simulink library "ddm"  (R2021b)
settings: Solver=VariableStepAuto  StartTime=0.0  StopTime=10.0  RelTol=1e-3
undefined symbols (not defined in the file): ADDM_FrTMTqDev_X_Nm, ADDM_RrTMTqDev_X_Nm, ENUM_ADASACCSTA_ERROR, ENUM_ADASACCSTA_OFF, ENUM_ADASACCSTA_STANDBY, ENUM_ALLOWMOV_ALLOWREADY, ENUM_APS, ENUM_BRKSTA_ERROR, ENUM_BRKSTA_OFF, ENUM_BRKSTA_ON, ENUM_BRKSW_INVALID, ENUM_BRKSW_OFF, ENUM_BRKSW_ON, ENUM_CHGPREACTERRSTA_OBCPRE, ENUM_DCDCFAULTSTA_ANYFAULTLV1, ENUM_DCDCFAULTSTA_ANYFAULTLV2, ENUM_DRIVETRAIN_AWD, ENUM_DRIVETRAIN_FWD, ENUM_DRIVETRAIN_RWD, ENUM_EDUDRTSTA_NORMAL, ENUM_EPBERROR_FAILED, ENUM_EPBSTA_APPLIED, ENUM_EPBSTA_RELEASED, ENUM_ESCAPSSta_APSUNAVAILABLE, ENUM_GEARACTUALPOSN_INVALID, ENUM_GEARACTUALPOSN_P, ENUM_HVBATTREADYPRE_READY, ENUM_HWRESETSTA_HWRESETING, ENUM_MCUWARN_LV0, ENUM_MCUWARN_LV1, ENUM_MCUWARN_LV2, ENUM_MCUWARN_LV3, ENUM_MCUWARN_NOERROR, ENUM_OBCFAULTSTA_ANYFAULT, ENUM_PAS_R2F2, ENUM_PDFAULT_BATTPDFAIL, ENUM_PDFAULT_DCDCDISABLE, ENUM_PDFAULT_MCUDISABLE, ENUM_PDFAULT_MCUDISCHRG, ENUM_POWERSTA_OFF, ENUM_POWERSTA_ON, ENUM_POWERSTA_READY, ENUM_POWERSTA_STANDBY, ENUM_PRESSINDI_LOW, ENUM_PUFAULT_BATTUPFAIL, ENUM_PUFAULT_DCDCENABLEFAIL, ENUM_PUFAULT_PRECHRGCHKFAIL, ENUM_PUFAULT_SAFETYCHKFAIL, ENUM_PWRSTASW_OFF, ENUM_PWRSTASW_OFFA, ENUM_PWRSTASW_OFFCHVCHRG, ENUM_PWRSTASW_OFFCLVCHRG, ENUM_PWRSTASW_ON, ENUM_PWRSTASW_ONHVCHRG, ENUM_PWRSTASW_READY, ENUM_PWRSTASW_STANDBY, ENUM_RAPSErrWarnSta_NORMAL, ENUM_RAPSErrWarnSta_RAPSERRLV1, ENUM_SHIFTCOMMAND_P, ENUM_SHIFTERERRSTA_PBUTTONFAILURE ... (+471)
libraries: hcu_lib x540, simulink x3
(part 26 of 26)

== system ddm/DDM/DDM/VMC_DDM/Zone_dr Error/Zone_dr Error  ==
  note: Diagnostics and Fault Handling
  note: Release Condiction After Decision
  note: Test Pass Criteria
  note: Test Detection Criteria
  task_time_s : Inport
  VDDM_DrVCUNoComCFS_flg : Inport  Port=2
  No_CAN4_BUS_OFF : Inport  Port=3
  VPMM_PowerSta_enum : Inport  Port=4
  VINP_ZoneDrMalfunLevel_enum : Inport  Port=5
  DTC_clear_request : Inport  Port=6
  Constant : Constant  Value=ENUM_POWERSTA_OFF
  Constant1 : Constant  Value=ENUM_POWERSTA_OFF
  Constant10 : Constant  Value=ZERO_INT
  Constant11 : Constant  Value=KDDM_VMCDiagnosisOffSW_flg
  Constant12 : Constant  Value=ENUM_POWERSTA_OFF
  Constant13 : Constant  Value=ENUM_POWERSTA_STANDBY
  Constant14 : Constant  Value=TRUE
  Constant15 : Constant  Value=FALSE
  Constant2 : Constant  Value=FALSE
  Constant3 : Constant  Value=ENUM_ZONEMALFUNLV_NORMAL
  Constant34 : Constant  Value=KDDM_ZoneDrSigErrDTC_cnt
  Constant4 : Constant  Value=KDDM_ZoneDrSigErrDetTO_s
  Constant5 : Constant  Value=TRUE
  Constant6 : Constant  Value=KDDM_ZoneDrSigErrPassTO_s
  Constant7 : Constant  Value=KDDM_ZoneDrSigErrDTC_cnt
  Constant8 : Constant  Value=ENUM_ZONEMALFUNLV_NORMAL
  Constant9 : Constant  Value=KDDM_ZoneDrSigErrPassTO_s
  DTC_Couter : hcu_lib/Basic_Blocks/DTC_Couter
  DTC_Info : hcu_lib/Basic_Blocks/DTC_Info
  Equal{,1..2,4} (4 alike) : RelationalOperator  Operator=~=  OutDataTypeStr=boolean  RndMeth=Simplest
  Equal3 : RelationalOperator  OutDataTypeStr=boolean  RndMeth=Simplest
  Equal6 : RelationalOperator  Operator===  OutDataTypeStr=boolean  RndMeth=Simplest
  Equal7 : RelationalOperator  Operator===  OutDataTypeStr=boolean  RndMeth=Simplest
  Logical Operator17 : Logic  Operator=NOT  AllPortsSameDT=off  OutDataTypeStr=boolean
  Logical Operator2 : Logic  Inputs=3  AllPortsSameDT=off  OutDataTypeStr=boolean
  Logical Operator21 : Logic  Operator=NOT  AllPortsSameDT=off  OutDataTypeStr=boolean
  Logical Operator23 : Logic  Inputs=3  AllPortsSameDT=off  OutDataTypeStr=boolean
  Logical Operator6 : Logic  Operator=NOT  AllPortsSameDT=off  OutDataTypeStr=boolean
  Logical Operator8 : Logic  Operator=OR  Inputs=4  AllPortsSameDT=off  OutDataTypeStr=boolean
  Logical Operator9 : Logic  AllPortsSameDT=off  OutDataTypeStr=boolean
  Relational Operator : RelationalOperator  Operator=>  OutDataTypeStr=boolean  RndMeth=Simplest
  Switch2 : Switch  Criteria=u2 ~= 0
  Switch3 : Switch  Criteria=u2 ~= 0
  Switch4 : Switch  Criteria=u2 ~= 0
  Terminator : Terminator
  Test Detection Criteria : hcu_lib/Basic_Blocks/Test Detection Criteria
  Timer1 : hcu_lib/Basic_Blocks/Timer
  Unit Delay2 : UnitDelay  SampleTime=-1  HasFrameUpgradeWarning=on
  VDDM_ZoneDrSigErrCFS_flg : Outport
  VDDM_ZoneDrSigErrDetDTC_raw32 : Outport  Port=2
  wires:
  DTC_Info/1 -> [VDDM_ZoneDrSigErrDetDTC_raw32]  "VDDM_ZoneDrSigErrDetDTC_raw32"
  [DTC_clear_request] -> DTC_Info/4
  [VDDM_ZoneDrSigErrCFS_flg] -> DTC_Info/3
  [VDDM_ZoneDrSigErrPass_flg] -> DTC_Info/2
  [VDDM_ZoneDrSigErrDet_flg] -> DTC_Info/1
  [VDDM_DrVCUNoComCFS_flg] -> Logical Operator21/1
  Equal1/1 -> Logical Operator23/3
  [VINP_ZoneDrMalfunLevel_enum] -> Equal2/1
  Constant11/1 -> Logical Operator8/4
  [VDDM_ZoneDrSigErrDetDTC_raw32] -> VDDM_ZoneDrSigErrDetDTC_raw32/1
  Constant10/1 -> Relational Operator/2
  [VINP_ZoneDrMalfunLevel_enum] -> Equal4/1
  Constant8/1 -> Equal4/2
  Switch2/1 -> Test Detection Criteria/1
  Equal4/1 -> Switch3/1
  Equal2/1 -> Switch2/1
  Constant3/1 -> Equal2/2
  DTC_Couter/1 -> [VDDM_ZoneDrSigErrCFS_flg]  "VDDM_ZoneDrSigErrCFS_flg"
  Relational Operator/1 -> Terminator/1  "VDDM_ZoneDrSigErrDFS_flg"
  [VDDM_ZoneDrSigErrDet_flg] -> DTC_Couter/1
  [VDDM_ZoneDrSigErrCFSRls_flg] -> DTC_Couter/2
  Constant34/1 -> DTC_Couter/3
  DTC_Couter/2 -> Relational Operator/1  "VDDM_ZoneDrSigErrDTC_cnt"
  Constant9/1 -> Timer1/4
  [task_time_s] -> Timer1/3
  Test Detection Criteria/1 -> [VDDM_ZoneDrSigErrDet_flg]  "VDDM_ZoneDrSigErrDet_flg"
  Constant7/1 -> Test Detection Criteria/3
  Constant4/1 -> Test Detection Criteria/4
  [task_time_s] -> Test Detection Criteria/2
  task_time_s/1 -> [task_time_s]  "task_time_s"
  Switch3/1 -> Timer1/2, Logical Operator6/1
  Constant1/1 -> Equal1/2
  [No_CAN4_BUS_OFF] -> Logical Operator23/1
  Logical Operator21/1 -> Logical Operator23/2
  Constant5/1 -> Switch3/3
  Logical Operator23/1 -> Switch3/2
  [VPMM_PowerSta_enum] -> Equal1/1
  Logical Operator17/1 -> Logical Operator2/2
  [VDDM_DrVCUNoComCFS_flg] -> Logical Operator17/1
  Equal/1 -> Logical Operator2/3
  VINP_ZoneDrMalfunLevel_enum/1 -> [VINP_ZoneDrMalfunLevel_enum]
  No_CAN4_BUS_OFF/1 -> [No_CAN4_BUS_OFF]
  VPMM_PowerSta_enum/1 -> [VPMM_PowerSta_enum]
  DTC_clear_request/1 -> [DTC_clear_request]
  VDDM_DrVCUNoComCFS_flg/1 -> [VDDM_DrVCUNoComCFS_flg]
  Timer1/1 -> Equal3/1
  [VPMM_PowerSta_enum] -> Equal/1
  Logical Operator8/1 -> Switch4/2
  [VPMM_PowerSta_enum] -> Equal7/1
  Constant14/1 -> Switch4/1
  Constant2/1 -> Switch2/3
  Constant12/1 -> Equal6/2
  Unit Delay2/1 -> Equal6/1
  Constant/1 -> Equal/2
  Constant13/1 -> Equal7/2
  Logical Operator6/1 -> Timer1/1
  Logical Operator2/1 -> Switch2/2
  [DTC_clear_request] -> Logical Operator8/3
  [VDDM_ZoneDrSigErrPass_flg] -> Logical Operator8/1
  [No_CAN4_BUS_OFF] -> Logical Operator2/1
  Switch4/1 -> [VDDM_ZoneDrSigErrCFSRls_flg]  "VDDM_ZoneDrSigErrCFSRls_flg"
  Logical Operator9/1 -> Logical Operator8/2
  [VPMM_PowerSta_enum] -> Unit Delay2/1
  Constant6/1 -> Equal3/2
  Equal7/1 -> Logical Operator9/2
  Equal6/1 -> Logical Operator9/1
  Constant15/1 -> Switch4/3
  [VDDM_ZoneDrSigErrCFS_flg] -> VDDM_ZoneDrSigErrCFS_flg/1
  Equal3/1 -> [VDDM_ZoneDrSigErrPass_flg]  "VDDM_ZoneDrSigErrPass_flg"

== system ddm/DDM/DDM/VMC_DDM/Zone_fr Error/Zone_fr Error  ==
  note: Test Detection Criteria
  note: Test Pass Criteria
  note: Release Condiction After Decision
  note: Diagnostics and Fault Handling
  task_time_s : Inport
  VDDM_FrVCUNoComCFS_flg : Inport  Port=2
  No_CAN4_BUS_OFF : Inport  Port=3
  VPMM_PowerSta_enum : Inport  Port=4
  ZoneFrMalfunLevel_enum : Inport  Port=5
  DTC_clear_request : Inport  Port=6
  Constant : Constant  Value=ENUM_POWERSTA_OFF
  Constant1 : Constant  Value=ENUM_POWERSTA_OFF
  Constant10 : Constant  Value=ZERO_INT
  Constant11 : Constant  Value=KDDM_VMCDiagnosisOffSW_flg
  Constant12 : Constant  Value=ENUM_POWERSTA_OFF
  Constant13 : Constant  Value=ENUM_POWERSTA_STANDBY
  Constant14 : Constant  Value=TRUE
  Constant15 : Constant  Value=FALSE
  Constant2 : Constant  Value=FALSE
  Constant3 : Constant  Value=ENUM_ZONEMALFUNLV_NORMAL
  Constant34 : Constant  Value=KDDM_ZoneFrSigErrDTC_cnt
  Constant4 : Constant  Value=KDDM_ZoneFrSigErrDetTO_s
  Constant5 : Constant  Value=TRUE
  Constant6 : Constant  Value=KDDM_ZoneFrSigErrPassTO_s
  Constant7 : Constant  Value=KDDM_ZoneFrSigErrDTC_cnt
  Constant8 : Constant  Value=ENUM_ZONEMALFUNLV_NORMAL
  Constant9 : Constant  Value=KDDM_ZoneFrSigErrPassTO_s
  DTC_Couter : hcu_lib/Basic_Blocks/DTC_Couter
  DTC_Info : hcu_lib/Basic_Blocks/DTC_Info
  Equal{,1..2,4} (4 alike) : RelationalOperator  Operator=~=  OutDataTypeStr=boolean  RndMeth=Simplest
  Equal3 : RelationalOperator  OutDataTypeStr=boolean  RndMeth=Simplest
  Equal6 : RelationalOperator  Operator===  OutDataTypeStr=boolean  RndMeth=Simplest
  Equal7 : RelationalOperator  Operator===  OutDataTypeStr=boolean  RndMeth=Simplest
  Logical Operator17 : Logic  Operator=NOT  AllPortsSameDT=off  OutDataTypeStr=boolean
  Logical Operator2 : Logic  Inputs=3  AllPortsSameDT=off  OutDataTypeStr=boolean
  Logical Operator21 : Logic  Operator=NOT  AllPortsSameDT=off  OutDataTypeStr=boolean
  Logical Operator23 : Logic  Inputs=3  AllPortsSameDT=off  OutDataTypeStr=boolean
  Logical Operator6 : Logic  Operator=NOT  AllPortsSameDT=off  OutDataTypeStr=boolean
  Logical Operator8 : Logic  Operator=OR  Inputs=4  AllPortsSameDT=off  OutDataTypeStr=boolean
  Logical Operator9 : Logic  AllPortsSameDT=off  OutDataTypeStr=boolean
  Relational Operator : RelationalOperator  Operator=>  OutDataTypeStr=boolean  RndMeth=Simplest
  Switch2 : Switch  Criteria=u2 ~= 0
  Switch3 : Switch  Criteria=u2 ~= 0
  Switch4 : Switch  Criteria=u2 ~= 0
  Terminator : Terminator
  Test Detection Criteria : hcu_lib/Basic_Blocks/Test Detection Criteria
  Timer1 : hcu_lib/Basic_Blocks/Timer
  Unit Delay2 : UnitDelay  SampleTime=-1  HasFrameUpgradeWarning=on
  VDDM_ZoneFrSigErrCFS_flg : Outport
  VDDM_ZoneFrSigErrDetDTC_raw32 : Outport  Port=2
  wires:
  DTC_Info/1 -> [VDDM_ZoneFrSigErrDetDTC_raw32]  "VDDM_ZoneFrSigErrDetDTC_raw32"
  [DTC_clear_request] -> DTC_Info/4
  [VDDM_ZoneFrSigErrCFS_flg] -> DTC_Info/3
  [VDDM_ZoneFrSigErrPass_flg] -> DTC_Info/2
  [VDDM_ZoneFrSigErrDet_flg] -> DTC_Info/1
  [VDDM_FrVCUNoComCFS_flg] -> Logical Operator17/1
  Equal3/1 -> [VDDM_ZoneFrSigErrPass_flg]  "VDDM_ZoneFrSigErrPass_flg"
  [VDDM_ZoneFrSigErrCFS_flg] -> VDDM_ZoneFrSigErrCFS_flg/1
  Constant15/1 -> Switch4/3
  Equal6/1 -> Logical Operator9/1
  Equal7/1 -> Logical Operator9/2
  Constant6/1 -> Equal3/2
  [VPMM_PowerSta_enum] -> Unit Delay2/1
  Logical Operator9/1 -> Logical Operator8/2
  Switch4/1 -> [VDDM_ZoneFrSigErrCFSRls_flg]  "VDDM_ZoneFrSigErrCFSRls_flg"
  [No_CAN4_BUS_OFF] -> Logical Operator2/1
  [VDDM_ZoneFrSigErrPass_flg] -> Logical Operator8/1
  [DTC_clear_request] -> Logical Operator8/3
  Logical Operator2/1 -> Switch2/2
  Logical Operator6/1 -> Timer1/1
  Constant13/1 -> Equal7/2
  Constant/1 -> Equal/2
  Unit Delay2/1 -> Equal6/1
  Constant12/1 -> Equal6/2
  Constant2/1 -> Switch2/3
  Constant14/1 -> Switch4/1
  [VPMM_PowerSta_enum] -> Equal7/1
  Logical Operator8/1 -> Switch4/2
  [VPMM_PowerSta_enum] -> Equal/1
  Timer1/1 -> Equal3/1
  VDDM_FrVCUNoComCFS_flg/1 -> [VDDM_FrVCUNoComCFS_flg]
  DTC_clear_request/1 -> [DTC_clear_request]
  VPMM_PowerSta_enum/1 -> [VPMM_PowerSta_enum]
  No_CAN4_BUS_OFF/1 -> [No_CAN4_BUS_OFF]
  ZoneFrMalfunLevel_enum/1 -> [ZoneFrMalfunLevel_enum]
  Equal/1 -> Logical Operator2/3
  Logical Operator17/1 -> Logical Operator2/2
  [VPMM_PowerSta_enum] -> Equal1/1
  Logical Operator23/1 -> Switch3/2
  Constant5/1 -> Switch3/3
  Logical Operator21/1 -> Logical Operator23/2
  [No_CAN4_BUS_OFF] -> Logical Operator23/1
  Constant1/1 -> Equal1/2
  Switch3/1 -> Logical Operator6/1, Timer1/2
  task_time_s/1 -> [task_time_s]  "task_time_s"
  [task_time_s] -> Test Detection Criteria/2
  Constant4/1 -> Test Detection Criteria/4
  Constant7/1 -> Test Detection Criteria/3
  Test Detection Criteria/1 -> [VDDM_ZoneFrSigErrDet_flg]  "VDDM_ZoneFrSigErrDet_flg"
  [task_time_s] -> Timer1/3
  Constant9/1 -> Timer1/4
  DTC_Couter/2 -> Relational Operator/1  "VDDM_ZoneFrSigErrDTC_cnt"
  Constant34/1 -> DTC_Couter/3
  [VDDM_ZoneFrSigErrCFSRls_flg] -> DTC_Couter/2
  [VDDM_ZoneFrSigErrDet_flg] -> DTC_Couter/1
  Relational Operator/1 -> Terminator/1  "VDDM_ZoneFrSigErrDFS_flg"
  DTC_Couter/1 -> [VDDM_ZoneFrSigErrCFS_flg]  "VDDM_ZoneFrSigErrCFS_flg"
  Constant3/1 -> Equal2/2
  Equal2/1 -> Switch2/1
  Equal4/1 -> Switch3/1
  Switch2/1 -> Test Detection Criteria/1
  Constant8/1 -> Equal4/2
  [ZoneFrMalfunLevel_enum] -> Equal4/1
  Constant10/1 -> Relational Operator/2
  [VDDM_ZoneFrSigErrDetDTC_raw32] -> VDDM_ZoneFrSigErrDetDTC_raw32/1
  Constant11/1 -> Logical Operator8/4
  [ZoneFrMalfunLevel_enum] -> Equal2/1
  Equal1/1 -> Logical Operator23/3
  [VDDM_FrVCUNoComCFS_flg] -> Logical Operator21/1

== system ddm/DDM/DDM/PMM/SW failure/Driver seat switch failure/Subsystem ==
  In1 : Inport
  Trigger : TriggerPort  VariantControl=Variant  PortDimensions=1
  Constant15 : Constant  Value=KDDM_DrStSW_s
  Logical Operator3 : Logic  Operator=NOT  AllPortsSameDT=off  OutDataTypeStr=boolean
  Relational Operator3 : RelationalOperator  Operator=<=  OutDataTypeStr=boolean  RndMeth=Simplest
  SR_Latch1 : hcu_lib/Basic_Blocks/SR_Latch
  Fault_flg : Outport
  wires:
  Logical Operator3/1 -> SR_Latch1/2
  SR_Latch1/1 -> Fault_flg/1
  In1/1 -> Relational Operator3/1
  Constant15/1 -> Relational Operator3/2
  Relational Operator3/1 -> SR_Latch1/1, Logical Operator3/1

== system ddm/DDM/DDM/PMM/SW failure/FL Door switch failure/Subsystem ==
  In1 : Inport
  Trigger : TriggerPort  VariantControl=Variant  PortDimensions=1
  Constant15 : Constant  Value=KDDM_FLDoorSW_s
  Logical Operator3 : Logic  Operator=NOT  AllPortsSameDT=off  OutDataTypeStr=boolean
  Relational Operator3 : RelationalOperator  Operator=<=  OutDataTypeStr=boolean  RndMeth=Simplest
  SR_Latch1 : hcu_lib/Basic_Blocks/SR_Latch
  Fault_flg : Outport
  wires:
  Logical Operator3/1 -> SR_Latch1/2
  SR_Latch1/1 -> Fault_flg/1
  In1/1 -> Relational Operator3/1
  Constant15/1 -> Relational Operator3/2
  Relational Operator3/1 -> SR_Latch1/1, Logical Operator3/1

== system ddm/DDM/DDM/PMM/SW failure/FR Door switch failure/Subsystem ==
  In1 : Inport
  Trigger : TriggerPort  VariantControl=Variant  PortDimensions=1
  Constant15 : Constant  Value=KDDM_FRDoorSW_s
  Logical Operator3 : Logic  Operator=NOT  AllPortsSameDT=off  OutDataTypeStr=boolean
  Relational Operator3 : RelationalOperator  Operator=<=  OutDataTypeStr=boolean  RndMeth=Simplest
  SR_Latch1 : hcu_lib/Basic_Blocks/SR_Latch
  Fault_flg : Outport
  wires:
  Logical Operator3/1 -> SR_Latch1/2
  SR_Latch1/1 -> Fault_flg/1
  In1/1 -> Relational Operator3/1
  Constant15/1 -> Relational Operator3/2
  Relational Operator3/1 -> SR_Latch1/1, Logical Operator3/1

== system ddm/DDM/DDM/PMM/SW failure/Hood switch failure/Subsystem ==
  In1 : Inport
  Trigger : TriggerPort  VariantControl=Variant  PortDimensions=1
  Constant15 : Constant  Value=KDDM_HoodSW_s
  Logical Operator3 : Logic  Operator=NOT  AllPortsSameDT=off  OutDataTypeStr=boolean
  Relational Operator3 : RelationalOperator  Operator=<=  OutDataTypeStr=boolean  RndMeth=Simplest
  SR_Latch1 : hcu_lib/Basic_Blocks/SR_Latch
  Fault_flg : Outport
  wires:
  Logical Operator3/1 -> SR_Latch1/2
  SR_Latch1/1 -> Fault_flg/1
  In1/1 -> Relational Operator3/1
  Constant15/1 -> Relational Operator3/2
  Relational Operator3/1 -> SR_Latch1/1, Logical Operator3/1

== system ddm/DDM/DDM/PMM/SW failure/RL Door switch failure/Subsystem ==
  In1 : Inport
  Trigger : TriggerPort  VariantControl=Variant  PortDimensions=1
  Constant15 : Constant  Value=KDDM_RLDoorSW_s
  Logical Operator3 : Logic  Operator=NOT  AllPortsSameDT=off  OutDataTypeStr=boolean
  Relational Operator3 : RelationalOperator  Operator=<=  OutDataTypeStr=boolean  RndMeth=Simplest
  SR_Latch1 : hcu_lib/Basic_Blocks/SR_Latch
  Fault_flg : Outport
  wires:
  Logical Operator3/1 -> SR_Latch1/2
  SR_Latch1/1 -> Fault_flg/1
  In1/1 -> Relational Operator3/1
  Constant15/1 -> Relational Operator3/2
  Relational Operator3/1 -> SR_Latch1/1, Logical Operator3/1

== system ddm/DDM/DDM/PMM/SW failure/RR Door switch failure/Subsystem ==
  In1 : Inport
  Trigger : TriggerPort  VariantControl=Variant  PortDimensions=1
  Constant15 : Constant  Value=KDDM_RRDoorSW_s
  Logical Operator3 : Logic  Operator=NOT  AllPortsSameDT=off  OutDataTypeStr=boolean
  Relational Operator3 : RelationalOperator  Operator=<=  OutDataTypeStr=boolean  RndMeth=Simplest
  SR_Latch1 : hcu_lib/Basic_Blocks/SR_Latch
  Fault_flg : Outport
  wires:
  Logical Operator3/1 -> SR_Latch1/2
  SR_Latch1/1 -> Fault_flg/1
  In1/1 -> Relational Operator3/1
  Constant15/1 -> Relational Operator3/2
  Relational Operator3/1 -> SR_Latch1/1, Logical Operator3/1

== system ddm/DDM/DDM/PMM/SW failure/Tailgate switch failure/Subsystem ==
  In1 : Inport
  Trigger : TriggerPort  VariantControl=Variant  PortDimensions=1
  Constant15 : Constant  Value=KDDM_TailgaSW_s
  Logical Operator3 : Logic  Operator=NOT  AllPortsSameDT=off  OutDataTypeStr=boolean
  Relational Operator3 : RelationalOperator  Operator=<=  OutDataTypeStr=boolean  RndMeth=Simplest
  SR_Latch1 : hcu_lib/Basic_Blocks/SR_Latch
  Fault_flg : Outport
  wires:
  Logical Operator3/1 -> SR_Latch1/2
  SR_Latch1/1 -> Fault_flg/1
  In1/1 -> Relational Operator3/1
  Constant15/1 -> Relational Operator3/2
  Relational Operator3/1 -> SR_Latch1/1, Logical Operator3/1

== stateflow chart ddm/DDM/DDM/Chart ==
  (default) -> (junction 3)
  (junction 3) -> (junction 5) [order 1] : [VDDM_Lv4ErrCFS_flg || ...
      |  ZoneFrMalfunLevel_enum == ENUM_ZONEMALFUNLV_4TH || ...
      |  ZoneDrMalfunLevel_enum == ENUM_ZONEMALFUNLV_4TH]
  (junction 3) -> (junction 9) [order 2]
  (junction 5) -> (junction 18) : {VDDM_VehMalfunLevel_enum = 4;
      |  %Warning_lamp = 1;
      |  %IVI_popup = 4;
      |  VDDM_limphome_enum = 4;
      |  VDDM_EmergencyPwrDown_flg = TRUE;}
  (junction 9) -> (junction 14) [order 1] : [VDDM_Lv3ErrCFS_flg || ...
      |  VDDM_MCUF1NoComCFS_flg || ...
      |  VDDM_MCUR1NoComCFS_flg || ...
      |  VDDM_MCUF1RCErrCFS_flg || ...
      |  VDDM_MCUR1RCErrCFS_flg || ...
      |  VDDM_MCUF1CSErrCFS_flg || ...
      |  VDDM_MCUR1CSErrCFS_flg || ...
      |  ZoneFrMalfunLevel_enum == ENUM_ZONEMALFUNLV_3RD || ...
      |  ZoneDrMalfunLevel_enum == ENUM_ZONEMALFUNLV_3RD]
      | % add20250602 MCUN change to MCU
      | % Delete Powerup and Powerdown diagnostic
      | % Delete20250524 VDDM_FrVCUNoComCFS_flg
  (junction 9) -> (junction 22) [order 2]
  (junction 14) -> (junction 19) : {VDDM_VehMalfunLevel_enum = 3;
      |  %Warning_lamp = 1;
      |  %IVI_popup = 3;
      |  VDDM_limphome_enum = 3;
      |  VDDM_EmergencyPwrDown_flg = FALSE;}
  (junction 22) -> (junction 24) [order 1] : [VDDM_C3BMS6RCCFS_flg || ...
      |  VDDM_C3BMS6CSCFS_flg || ...
      |  VDDM_C3BMS6LCCFS_flg || ...
      |  VDDM_Lv2ErrCFS_flg || ...
      |  VDDM_BrkSWNoBacCFS_flg || ...
      |  VDDM_ESC1NoComCFS_flg || ...
      |  VDDM_ESC5NoComCFS_flg || ...
      |  VDDM_ESC1RCErrCFS_flg || ...
      |  VDDM_ESC5RCErrCFS_flg || ...
      |  VDDM_ESC1CSErrCFS_flg || ...
      |  VDDM_ESC5CSErrCFS_flg || ...
      |  VDDM_5vAPS1OoRCFS_flg || ...
      |  VDDM_5vAPS2OoRCFS_flg || ...
      |  VDDM_APS1SigOoRCFS_flg || ...
      |  VDDM_APS2SigOoRCFS_flg || ...
      |  VDDM_APSCorrErrCFS_flg || ...
      |  VDDM_DrVCUNoComCFS_flg ||...
      |  VDDM_FrMCUTqErrCFS_flg ||...
      |  VDDM_RrMCUTqErrCFS_flg ||...
      |  ZoneFrMalfunLevel_enum == ENUM_ZONEMALFUNLV_2ND || ...
      |  ZoneDrMalfunLevel_enum == ENUM_ZONEMALFUNLV_2ND ||...
      |  VDDM_C3BMS1RCCFS_flg || ...
      |  VDDM_C3BMS1CSCFS_flg || ...
      |  VDDM_C3BMS1LCCFS_flg || ...
      |  VDDM_FrVCUNoComCFS_flg]
      | % add20250515  BMS1LC,RC,CS
      | % add20250524 VDDM_FrVCUNoComCFS_flg
      | %Delete VDDM_ESCSigErrCFS_flg
      | % Delete20250516 CCU1,CCU2LC,RC,CS
      | % Delete20250519 VDDM_IniLVLoCFS_flg
      | % Delete20250522 VDDM_LVSupHiCFS_flg,VDDM_LVSupHiCFS_flg
  (junction 22) -> (junction 29) [order 2]
  (junction 24) -> (junction 26) : {VDDM_VehMalfunLevel_enum = 2;
      |  %Warning_lamp = 1;
      |  %IVI_popup = 2;
      |  VDDM_limphome_enum = 2;
      |  VDDM_EmergencyPwrDown_flg = FALSE;}
  (junction 29) -> (junction 31) [order 1] : [VDDM_C1ABM1RCCFS_flg || ...
      |  VDDM_C1ABM1CSCFS_flg || ...
      |  VDDM_C1ABM1LCCFS_flg || ...
      |  VDDM_Lv1ErrCFS_flg || ...
      |  VDDM_RrMCUDisCFS_flg || ...
      |  VDDM_FrMCUDisCFS_flg || ...
      |  VDDM_DCDCDisCFS_flg || ...
      |  VDDM_OBC4PreCFS_flg || ...
      |  VDDM_BrkSWErrCFS_flg || ...
      |  VDDM_DrStSWCFS_flg || ...
      |  VDDM_FLDoorSWCFS_flg || ...
      |  VDDM_FRDoorSWCFS_flg || ...
      |  VDDM_RLDoorSWCFS_flg || ...
      |  VDDM_RRDoorSWCFS_flg || ...
      |  VDDM_HoodSWCFS_flg || ...
      |  VDDM_TailgaSWCFS_flg || ...
      |  VDDM_KeyAuthCFS_flg || ...
      |  VDDM_LVInErrCFS_flg ||...
      |  VDDM_ONtoRdyCFS_flg || ...
      |  VDDM_Shifter1NoComCFS_flg || ...
      |  VDDM_Shifter1RCErrCFS_flg || ...
      |  VDDM_Shifter1CSErrCFS_flg || ...
      |  VDDM_EPBLockTOCFS_flg || ...
      |  VDDM_EPBUnlockTOCFS_flg || ...
      |  VDDM_FCM1NoComCFS_flg || ...
      |  VDDM_FCM1RCErrCFS_flg || ...
      |  VDDM_FCM1CSErrCFS_flg || ...
      |  VDDM_BMSSigErrCFS_flg ||...
      |  VDDM_FCMACCSigErrCFS_flg ||...
      |  VDDM_CCUSigErrCFS_flg ||...
      |  VDDM_ACCAccelCmdErrCFS_flg ||...
      |  VDDM_ShifterSigErrCFS_flg ||...
      |  VDDM_ZoneDrSigErrCFS_flg ||...
      |  VDDM_ZoneFrSigErrCFS_flg ||...
      |  VDDM_EPS1NoComCFS_flg ||...
      |  VDDM_EPS1RCErrCFS_flg ||...
      |  VDDM_EPS1CSErrCFS_flg ||...
      |  VDDM_EPSSigErrCFS_flg ||...
      |  VDDM_FrMCUSigErrCFS_flg ||...
      |  VDDM_RrMCUSigErrCFS_flg ||...
      |  VDDM_EPB1NoComCFS_flg ||...
      |  VDDM_EPB1RCErrCFS_flg ||...
      |  VDDM_EPB1CSErrCFS_flg ||...
      |  VDDM_EPBSigErrCFS_flg || ...
      |  ZoneFrMalfunLevel_enum == ENUM_ZONEMALFUNLV_1ST || ...
      |  ZoneDrMalfunLevel_enum == ENUM_ZONEMALFUNLV_1ST|| ...
      |  VDDM_RegenErrCFS_flg || ...
      |  VDDM_ESCSigErrCFS_flg || ...
      |  VDDM_HVB4PreCFS_flg || ...
      |  VDDM_FrMCU4PreCFS_flg || ...
      |  VDDM_RrMCU4PreCFS_flg ||...
      |  VDDM_DCDC4PreCFS_flg || ...
      |  VDDM_HVRlyCloCFS_flg || ...
      |  VDDM_BMSRdyCFS_flg || ...
      |  VDDM_DCDCEnaCFS_flg || ...
      |  VDDM_HiLvSaChkCFS_flg || ...
      |  VDDM_MidLvSaChkCFS_flg || ...
      |  VDDM_HVRlyOpCFS_flg || ...
      |  VDDM_RrMCUActCFS_flg || ...
      |  VDDM_FrMCUActCFS_flg ||...
      |  VDDM_C3CCU1RCCFS_flg || ...
      |  VDDM_C3CCU1CSCFS_flg || ...
      |  VDDM_C3CCU1LCCFS_flg || ...
      |  VDDM_C3CCU2RCCFS_flg || ...
      |  VDDM_C3CCU2CSCFS_flg || ...
      |  VDDM_C3CCU2LCCFS_flg ||...
      |  VDDM_IniLVLoCFS_flg ||...
      |  VDDM_LVSupLoCFS_flg || ...
      |  VDDM_LVSupHiCFS_flg]
      | %add20250218 VDDM_FrMCUDisCFS_flg
      | %add20250505 VDDM_RegenErrCFS_flg
      | %add20250512 VDDM_ESCSigErrCFS_flg
      | %add20250515 add Powerup and Powerdown diagnostic
      | %add20250516 add CCU1 、CCU2,LC,RC,CS
      | %add20250522 VDDM_IniLVLoCFS_flg,VDDM_LVSupHiCFS_flg,VDDM_LVSupHiCFS_flg]
      | %add20250602 VDDM_RegenErrCFS_flg
  (junction 29) -> (junction 36) [order 2] : {VDDM_VehMalfunLevel_enum = 0;
      |  %Warning_lamp = 0;
      |  %IVI_popup = 0;
      |  VDDM_limphome_enum = 0;
      |  VDDM_EmergencyPwrDown_flg = FALSE;}
  (junction 31) -> (junction 33) : {VDDM_VehMalfunLevel_enum = 1;
      |  %Warning_lamp = 0;
      |  %IVI_popup = 0;
      |  VDDM_limphome_enum = 0;
      |  VDDM_EmergencyPwrDown_flg = FALSE;}
  (junction 33) -> (junction 36)
  (junction 26) -> (junction 33)
  (junction 19) -> (junction 26)
  (junction 18) -> (junction 19)
  data: VDDM_Lv4ErrCFS_flg input; VDDM_5vAPS1OoRCFS_flg input; VDDM_5vAPS2OoRCFS_flg input; VDDM_BMSRdyCFS_flg input; VDDM_BrkSWErrCFS_flg input; VDDM_BrkSWNoBacCFS_flg input; VDDM_C1ABM1CSCFS_flg input; VDDM_C1ABM1LCCFS_flg input; VDDM_C1ABM1RCCFS_flg input; VDDM_C3BMS1CSCFS_flg input; VDDM_C3BMS1LCCFS_flg input; VDDM_C3BMS1RCCFS_flg input; VDDM_C3BMS6CSCFS_flg input; VDDM_C3BMS6LCCFS_flg input; VDDM_C3BMS6RCCFS_flg input; VDDM_C3CCU1CSCFS_flg input; VDDM_C3CCU1LCCFS_flg input; VDDM_C3CCU1RCCFS_flg input; VDDM_C3CCU2CSCFS_flg input; VDDM_C3CCU2LCCFS_flg input; VDDM_C3CCU2RCCFS_flg input; VDDM_DCDC4PreCFS_flg input; VDDM_DCDCDisCFS_flg input; VDDM_DCDCEnaCFS_flg input; VDDM_DrStSWCFS_flg input; VDDM_EPBLockTOCFS_flg input; VDDM_EPBUnlockTOCFS_flg input; VDDM_ESC1CSErrCFS_flg input; VDDM_ESC1NoComCFS_flg input; VDDM_ESC1RCErrCFS_flg input; VDDM_ESC5CSErrCFS_flg input; VDDM_ESC5NoComCFS_flg input; VDDM_ESC5RCErrCFS_flg input; VDDM_FLDoorSWCFS_flg input; VDDM_FRDoorSWCFS_flg input; VDDM_HVB4PreCFS_flg input; VDDM_HVRlyCloCFS_flg input; VDDM_HVRlyOpCFS_flg input; VDDM_HiLvSaChkCFS_flg input; VDDM_IniLVLoCFS_flg input; VDDM_KeyAuthCFS_flg input; VDDM_LVInErrCFS_flg input; VDDM_LVSupHiCFS_flg input; VDDM_LVSupLoCFS_flg input; VDDM_Lv1ErrCFS_flg input; VDDM_Lv2ErrCFS_flg input; VDDM_Lv3ErrCFS_flg input; VDDM_RrMCU4PreCFS_flg input; VDDM_RrMCUActCFS_flg input; VDDM_RrMCUDisCFS_flg input; VDDM_MCUF1CSErrCFS_flg input; VDDM_MCUF1NoComCFS_flg input; VDDM_MCUF1RCErrCFS_flg input; VDDM_MCUR1CSErrCFS_flg input; VDDM_MCUR1NoComCFS_flg input; VDDM_MCUR1RCErrCFS_flg input; VDDM_MidLvSaChkCFS_flg input; VDDM_OBC4PreCFS_flg input; VDDM_ONtoRdyCFS_flg input; VDDM_RLDoorSWCFS_flg input; VDDM_RRDoorSWCFS_flg input; VDDM_Shifter1CSErrCFS_flg input; VDDM_Shifter1NoComCFS_flg input; VDDM_Shifter1RCErrCFS_flg input; VDDM_VehMalfunLevel_enum output uint8; VDDM_EmergencyPwrDown_flg output boolean; VDDM_limphome_enum output uint8; VDDM_HoodSWCFS_flg input; VDDM_TailgaSWCFS_flg input; ZoneDrMalfunLevel_enum input; ZoneFrMalfunLevel_enum input; ENUM_ZONEMALFUNLV_1ST parameter; ENUM_ZONEMALFUNLV_2ND parameter; ENUM_ZONEMALFUNLV_3RD parameter; ENUM_ZONEMALFUNLV_4TH parameter; FALSE parameter; TRUE parameter; VDDM_APS1SigOoRCFS_flg input; VDDM_APS2SigOoRCFS_flg input; VDDM_APSCorrErrCFS_flg input; VDDM_FCM1NoComCFS_flg input; VDDM_FCM1RCErrCFS_flg input; VDDM_FCM1CSErrCFS_flg input; VDDM_BMSSigErrCFS_flg input; VDDM_FCMACCSigErrCFS_flg input; VDDM_CCUSigErrCFS_flg input; VDDM_ACCAccelCmdErrCFS_flg input; VDDM_ESCSigErrCFS_flg input; VDDM_ShifterSigErrCFS_flg input; VDDM_DrVCUNoComCFS_flg input; VDDM_FrVCUNoComCFS_flg input; VDDM_ZoneDrSigErrCFS_flg input; VDDM_ZoneFrSigErrCFS_flg input; VDDM_EPS1NoComCFS_flg input; VDDM_EPS1RCErrCFS_flg input; VDDM_EPS1CSErrCFS_flg input; VDDM_EPSSigErrCFS_flg input; VDDM_FrMCUSigErrCFS_flg input; VDDM_RrMCUSigErrCFS_flg input; VDDM_EPB1NoComCFS_flg input; VDDM_EPB1RCErrCFS_flg input; VDDM_EPB1CSErrCFS_flg input; VDDM_EPBSigErrCFS_flg input; VDDM_FrMCUTqErrCFS_flg input; VDDM_RrMCUTqErrCFS_flg input; VDDM_FrMCU4PreCFS_flg input; VDDM_FrMCUDisCFS_flg input; VDDM_FrMCUActCFS_flg input; VDDM_RegenErrCFS_flg input
